simulink model "cau53b"  (R2015a)
settings: Solver=ode45  StartTime=0.0  StopTime=5  RelTol=1e-3
libraries: dspsrcs4 x4, commfilt2 x2, dspstat3 x1, commchan3 x1, commsink2 x1, commutil2 x1, commrandsrc2 x1
settings Model: Creator=Ming Duc  LastModifiedBy=XUAN

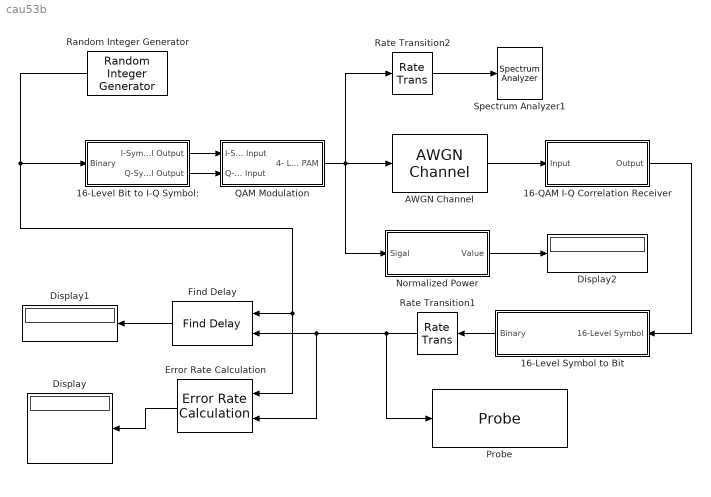
== system cau53b ==
  " Normalized Power" : Subsystem
  16-Level Bit to I-Q Symbol: : Subsystem
  16-Level Symbol to Bit : Subsystem
  16-QAM I-Q Correlation Receiver : Subsystem
  AWGN Channel : commchan3/AWGN Channel  InputProcessing=Columns as channels (frame based)  seed=67  noiseMode="Signal to noise ratio  (Eb/No)"  EbNodB=12  EsNodB=10  SNRdB=10  bitsPerSym=1  Ps=1  Tsym=1  variance=1
  Display : Display
  Display1 : Display
  Display2 : Display
  Error Rate Calculation : commsink2/Error Rate Calculation  N=0  st_delay=0  cp_mode=Select samples from mask  subframe=1  PMode=Port  WsName=ErrorVec  RsMode2=off  stop=off  numErr=100  maxBits=1e6
  Find Delay : commutil2/Find Delay  corrLength=200  chgSigOP=off  stopUpdate=off  numConstDelay=3
  Probe : Probe  ProbeWidth=off  ProbeComplexSignal=off  ProbeSignalDimensions=on
  QAM Modulation : Subsystem
  Random Integer Generator : commrandsrc2/Random Integer Generator  mul=8  seed=67  Ts=1/1000  frameBased=off  sampPerFrame=1  orient=off  outDataType=double
  Rate Transition1 : RateTransition  OutPortSampleTime=2e-5
  Rate Transition2 : RateTransition  OutPortSampleTime=2e-5
  Spectrum Analyzer1 : SpectrumAnalyzer
  wires:
  Random Integer Generator/1 -> Error Rate Calculation/1, Find Delay/1, 16-Level Bit to I-Q Symbol:/1(Binary)
  16-Level Symbol to Bit/1(Binary) -> Rate Transition1/1
  Find Delay/1 -> Display1/1
  Error Rate Calculation/1 -> Display/1
  " Normalized Power"/1(Value) -> Display2/1
  AWGN Channel/1 -> 16-QAM I-Q Correlation Receiver/1(Input)
  16-QAM I-Q Correlation Receiver/1(Output) -> 16-Level Symbol to Bit/1(16-Level Symbol)
  Rate Transition2/1 -> Spectrum Analyzer1/1
  QAM Modulation/1(4- Level PAM) -> Rate Transition2/1, " Normalized Power"/1(Sigal), AWGN Channel/1
  Rate Transition1/1 -> Probe/1, Error Rate Calculation/2, Find Delay/2
  16-Level Bit to I-Q Symbol:/2(Q-Symbol Output) -> QAM Modulation/2(Q-Symbol Input)
  16-Level Bit to I-Q Symbol:/1(I-Symbol Output) -> QAM Modulation/1(I-Symbol Input)

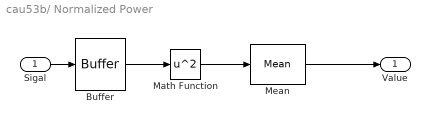
== system cau53b/ Normalized Power ==
  Sigal : Inport
  Buffer : Buffer  TreatMby1Signals=One channel
  Math Function : Math  Operator=square  SaturateOnIntegerOverflow=on
  Mean : dspstat3/Mean  run=off  reset_popup=None  InputProcessing=Columns as channels (frame based)  directionMode=Each column  dimension=1  treatSBRowAsCol=off  roiEnable=off  roiType=Rectangles  roiPortion=Entire ROI  roiOutput=Individual statistics for each ROI  roiFlag=off  outputDataTypeStr=Inherit: Same as accumulator  outputLastDataTypeStr=Inherit: Same as accumulator  outputMin=[]  outputMax=[]  roundingMode=Floor  overflowMode=off
  Value : Outport
  wires:
  Sigal/1 -> Buffer/1
  Buffer/1 -> Math Function/1
  Math Function/1 -> Mean/1
  Mean/1 -> Value/1

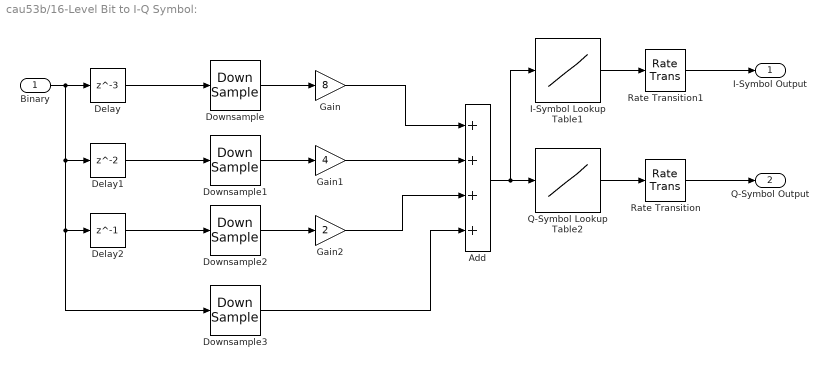
== system cau53b/16-Level Bit to I-Q Symbol: ==
  Binary : Inport
  Add : Sum  Inputs=++++
  Delay : Delay  DelayLength=3  InitialCondition=0
  Delay1 : Delay  InitialCondition=0
  Delay2 : Delay  DelayLength=1  InitialCondition=0
  Downsample{,1..3} (4 alike) : DownSample  N=4  RateOptions=Allow multirate processing
  Gain : Gain  Gain=8
  Gain1 : Gain  Gain=4
  Gain2 : Gain  Gain=2
  I-Symbol Lookup Table1 : Lookup_n-D  NumberOfTableDimensions=1  BreakpointsForDimension1=[0,1,2,3,4,5,6,7,8,9,10,11,12,13,14,15]  Table=[-1,-3,-1,-3,1,3,1,3,-1,-3,-1,-3,1,3,1,3]  InternalRulePriority=Speed  RndMeth=Simplest  InputSameDT=on
  Q-Symbol Lookup Table2 : Lookup_n-D  NumberOfTableDimensions=1  BreakpointsForDimension1=[0,1,2,3,4,5,6,7,8,9,10,11,12,13,14,15]  Table=[1,1,3,3,1,1,3,3,-1,-1,-3,-3,-1,-1,-3,-3]  InternalRulePriority=Speed  RndMeth=Simplest  InputSameDT=on
  Rate Transition : RateTransition  OutPortSampleTime=2e-5
  Rate Transition1 : RateTransition  OutPortSampleTime=2e-5
  I-Symbol Output : Outport
  Q-Symbol Output : Outport  Port=2
  wires:
  Delay/1 -> Downsample/1
  Downsample/1 -> Gain/1
  Gain/1 -> Add/1
  Binary/1 -> Downsample3/1, Delay2/1, Delay1/1, Delay/1
  Downsample3/1 -> Add/4
  Gain2/1 -> Add/3
  Gain1/1 -> Add/2
  Delay1/1 -> Downsample1/1
  Delay2/1 -> Downsample2/1
  Add/1 -> I-Symbol Lookup Table1/1, Q-Symbol Lookup Table2/1
  Rate Transition/1 -> Q-Symbol Output/1
  Rate Transition1/1 -> I-Symbol Output/1
  Downsample2/1 -> Gain2/1
  Downsample1/1 -> Gain1/1
  Q-Symbol Lookup Table2/1 -> Rate Transition/1
  I-Symbol Lookup Table1/1 -> Rate Transition1/1

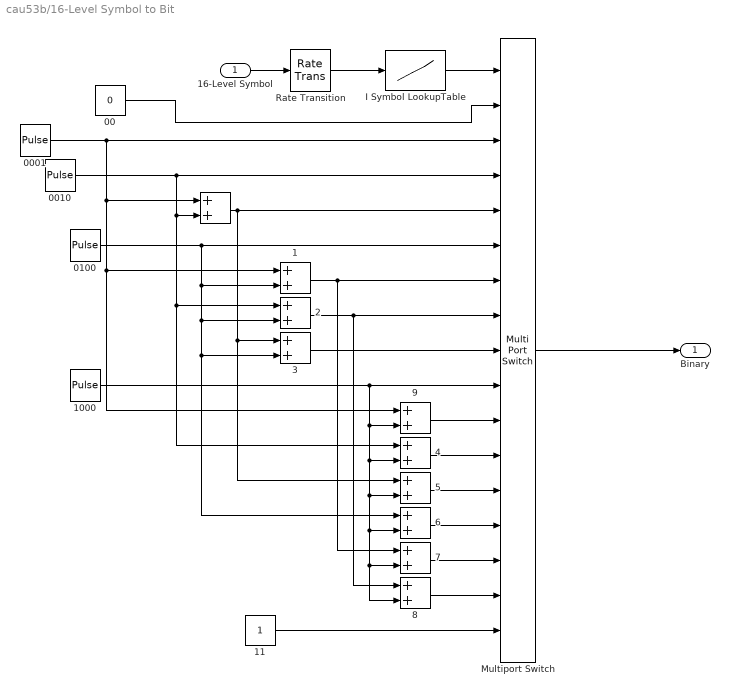
== system cau53b/16-Level Symbol to Bit ==
  16-Level Symbol : Inport
   {,1..9} (10 alike) : Sum
  00 : Constant  Value=0
  0001 : DiscretePulseGenerator  Amplitude=4  Period=10  PulseWidth=5  SampleTime=1/1000
  0010 : DiscretePulseGenerator  Amplitude=4  Period=10  PulseWidth=5  PhaseDelay=2  SampleTime=1/1000
  0100 : DiscretePulseGenerator  Amplitude=4  Period=10  PulseWidth=5  PhaseDelay=2  SampleTime=1/1000
  1000 : DiscretePulseGenerator  Amplitude=4  Period=10  PulseWidth=5  PhaseDelay=2  SampleTime=1/1000
  11 : Constant
  I Symbol LookupTable : Lookup_n-D  NumberOfTableDimensions=1  BreakpointsForDimension1=[-5:5]  Table=tanh([-5:5])  InternalRulePriority=Speed  RndMeth=Simplest  InputSameDT=on
  Multiport Switch : MultiPortSwitch  Inputs=16  DiagnosticForDefault=None
  Rate Transition : RateTransition
  Binary : Outport
  wires:
  16-Level Symbol/1 -> Rate Transition/1
  Multiport Switch/1 -> Binary/1
  Rate Transition/1 -> I Symbol LookupTable/1
  I Symbol LookupTable/1 -> Multiport Switch/1
  11/1 -> Multiport Switch/17
  00/1 -> Multiport Switch/2
  0001/1 -> " "/1, " 1"/1, " 9"/1, Multiport Switch/3
  " 1"/1 -> Multiport Switch/7, " 7"/1
  " 2"/1 -> Multiport Switch/8, " 8"/1
  " 8"/1 -> Multiport Switch/16
  " 7"/1 -> Multiport Switch/15
  " 6"/1 -> Multiport Switch/14
  " 5"/1 -> Multiport Switch/13
  " 4"/1 -> Multiport Switch/12
  0100/1 -> " 6"/1, " 3"/2, " 2"/2, " 1"/2, Multiport Switch/6
  " "/1 -> Multiport Switch/5, " 3"/1, " 5"/1
  " 3"/1 -> Multiport Switch/9
  " 9"/1 -> Multiport Switch/11
  1000/1 -> Multiport Switch/10, " 9"/2, " 8"/2, " 7"/2, " 6"/2, " 5"/2, " 4"/2
  0010/1 -> " "/2, " 2"/1, " 4"/1, Multiport Switch/4

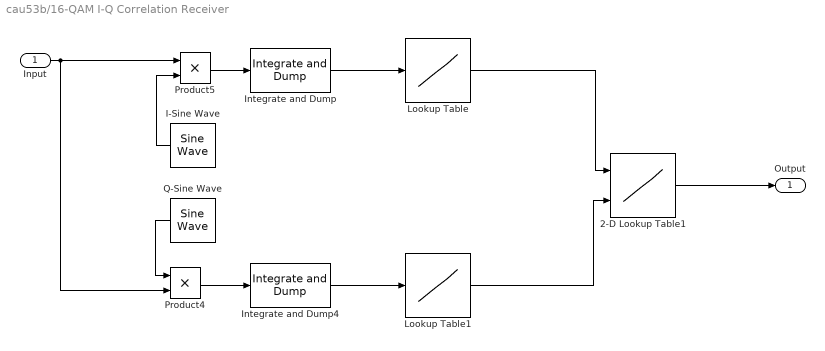
== system cau53b/16-QAM I-Q Correlation Receiver ==
  Input : Inport
  " Lookup Table" : Lookup_n-D  NumberOfTableDimensions=1  BreakpointsForDimension1=[-5:5]  Table=tanh([-5:5])  InternalRulePriority=Speed  RndMeth=Simplest  InputSameDT=on
  " Lookup Table1" : Lookup_n-D  NumberOfTableDimensions=1  BreakpointsForDimension1=[-5:5]  Table=tanh([-5:5])  InternalRulePriority=Speed  RndMeth=Simplest  InputSameDT=on
  2-D Lookup Table1 : Lookup_n-D  BreakpointsForDimension1=[1,2,3,4,5,6,7,8,9,10,11,12,13,14,15,16]  BreakpointsForDimension2=[1,2]  Table=reshape([-1,-3,-1,-3,1,3,1,3,-1,-3,-1,-3,1,3,1,3,1,1,3,3,1,1,3,3,-1,-1,-3,-3,-1,-1,-3,-3],16,2)  InternalRulePriority=Speed  RndMeth=Simplest  InputSameDT=on
  I-Sine Wave : dspsrcs4/Sine Wave  Amplitude=1  Frequency=100  Phase=0  SampleMode=Discrete  OutComplex=Real  CompMethod=Trigonometric fcn  TableSize=Speed  SampleTime=1/1000  SamplesPerFrame=1  ResetState=Restart at time zero  dataType=double  wordLen=16  udDataType=sfix(16)  fracBitsMode=Best precision  numFracBits=15  OutDataTypeStr=double  LastOutDataTypeStr=double
  Integrate and Dump : commfilt2/Integrate and Dump  obssamples=8  offsetsamples=0  nodump=off  roundingMode=Floor  overflowMode=off
  Integrate and Dump4 : commfilt2/Integrate and Dump  obssamples=8  offsetsamples=0  nodump=off  roundingMode=Floor  overflowMode=off
  Product4 : Product
  Product5 : Product
  Q-Sine Wave : dspsrcs4/Sine Wave  Amplitude=1  Frequency=100  Phase=0  SampleMode=Discrete  OutComplex=Real  CompMethod=Trigonometric fcn  TableSize=Speed  SampleTime=1/1000  SamplesPerFrame=1  ResetState=Restart at time zero  dataType=double  wordLen=16  udDataType=sfix(16)  fracBitsMode=Best precision  numFracBits=15  OutDataTypeStr=double  LastOutDataTypeStr=double
  Output : Outport
  wires:
  I-Sine Wave/1 -> Product5/2
  Q-Sine Wave/1 -> Product4/1
  Product5/1 -> Integrate and Dump/1
  Product4/1 -> Integrate and Dump4/1
  Input/1 -> Product4/2, Product5/1
  Integrate and Dump/1 -> " Lookup Table"/1
  Integrate and Dump4/1 -> " Lookup Table1"/1
  " Lookup Table"/1 -> 2-D Lookup Table1/1
  " Lookup Table1"/1 -> 2-D Lookup Table1/2
  2-D Lookup Table1/1 -> Output/1

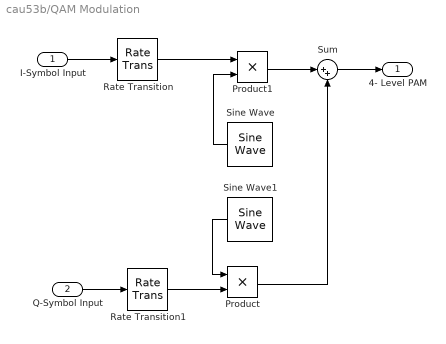
== system cau53b/QAM Modulation ==
  I-Symbol Input : Inport
  Q-Symbol Input : Inport  Port=2
  Product : Product
  Product1 : Product
  Rate Transition : RateTransition
  Rate Transition1 : RateTransition
  Sine Wave : dspsrcs4/Sine Wave  Amplitude=1  Frequency=100  Phase=0  SampleMode=Discrete  OutComplex=Real  CompMethod=Trigonometric fcn  TableSize=Speed  SampleTime=1/1000  SamplesPerFrame=1  ResetState=Restart at time zero  dataType=double  wordLen=16  udDataType=sfix(16)  fracBitsMode=Best precision  numFracBits=15  OutDataTypeStr=double  LastOutDataTypeStr=double
  Sine Wave1 : dspsrcs4/Sine Wave  Amplitude=1  Frequency=100  Phase=0  SampleMode=Discrete  OutComplex=Real  CompMethod=Trigonometric fcn  TableSize=Speed  SampleTime=1/1000  SamplesPerFrame=1  ResetState=Restart at time zero  dataType=double  wordLen=16  udDataType=sfix(16)  fracBitsMode=Best precision  numFracBits=15  OutDataTypeStr=double  LastOutDataTypeStr=double
  Sum : Sum  Inputs=|++
  4- Level PAM : Outport
  wires:
  Sine Wave/1 -> Product1/2
  Sine Wave1/1 -> Product/1
  Product1/1 -> Sum/1
  Product/1 -> Sum/2
  Sum/1 -> 4- Level PAM/1
  Q-Symbol Input/1 -> Rate Transition1/1
  Rate Transition1/1 -> Product/2
  I-Symbol Input/1 -> Rate Transition/1
  Rate Transition/1 -> Product1/1
